simulink model "gm_uz_pmsm_model_6LUT_pd_vnl"  (R2023a)
settings: Solver=FixedStepAuto  StartTime=0.0  StopTime=0.05  RelTol=1e-3
PreLoadFcn:
  | uz_pmsm_model_init_parameter
PostLoadFcn:
  | % Import the data from Excel for a lookup table
  | FluxMapData = readtable('C:\Users\Philipp\ultrazohm\ultrazohm_sw\ip_cores\uz_pmsm_model\FluxMapData_2023-05-26_13-07-57.csv');
  | % Row indices for lookup table
  | d_current_in_d_axis = FluxMapData(8:27,1:end);
  | % Column indices for lookup table
  | q_current_in_d_axis = FluxMapData(29:48,1:end);
  | % Output values for lookup table
  | d_Flux_d_axis = FluxMapData(50:69,1:end);
undefined symbols (not defined in the file or in its folder): d_current_d_Flux, d_current_q_Flux, entkopplung_dynamic, entkopplung_linear, entkopplung_static, Flux_d, Flux_q, friction_coefficient, inertia, k_i_d, k_p_d, k_p_q, Ki_Bo_d, Ki_Bo_q, Kp_Bo_d, Kp_Bo_q, L_d, L_q, Ldd, Ldq, Lqd, Lqq, parameter_nachfuerung, polepair, praediktion_entkopplung_nonlinear, psi_pm, q_current_d_Flux, q_current_q_Flux, R_1, simulate_mechanical, simulate_nonlinear_modell, simulate_open_loop, static_friction_torque, tau_sum, ts, ts_regler
libraries: hdlmdlgenlib x5, slpidlib x4, simulink x2
(part 2 of 2)

== system gm_uz_pmsm_model_6LUT_pd_vnl/uz_pmsm_model_6LUT_vnl ==
  reset_integrators : Inport
  simulate_mechanical : Inport  Port=2
  reciprocal_J : Inport  Port=3
  mu : Inport  Port=4
  M_n0 : Inport  Port=5
  R1 : Inport  Port=6
  polepairs : Inport  Port=7
  inputs : Inport  Port=8
  Data Type Conversion{11,15..17} (4 alike) : DataTypeConversion  OutDataTypeStr=single  RndMeth=Nearest  SaturateOnIntegerOverflow=off
  Demux : Demux
  Mux : Mux
  Switch : Switch  Criteria=u2 ~= 0  SaturateOnIntegerOverflow=off  InputSameDT=off
  Switch1 : Switch  Criteria=u2 ~= 0  SaturateOnIntegerOverflow=off  InputSameDT=off
  mechanical_system : Subsystem
  pmsm : Subsystem
  torque_calculation : Subsystem
  outputs : Outport
  wires:
  Mux/1 -> outputs/1
  inputs/1 -> Demux/1
  Data Type Conversion11/1 -> Mux/1
  Data Type Conversion15/1 -> Mux/2  "i_q"
  Data Type Conversion16/1 -> Mux/3  "i_q"
  Data Type Conversion17/1 -> Mux/4  "i_q"
  pmsm/1(I_d1) -> torque_calculation/1(I_d), Data Type Conversion11/1  "i_d"
  pmsm/4(I_q1) -> Data Type Conversion15/1, torque_calculation/5(I_q)  "i_q"
  mechanical_system/1(omega_mech) -> Switch1/1, Switch/1
  Demux/2 -> pmsm/3(u_q1)  "u_q"
  M_n0/1 -> mechanical_system/4(M_n0)
  torque_calculation/1(M_Mi) -> Data Type Conversion16/1, mechanical_system/2(M_Mi)
  reciprocal_J/1 -> mechanical_system/5(reciprocal_J)
  simulate_mechanical/1 -> Switch/2, Switch1/2
  mu/1 -> mechanical_system/3(mu)
  Demux/1 -> pmsm/2(u_d1)  "u_d"
  polepairs/1 -> torque_calculation/4(polepairs), pmsm/5(polepairs1)
  pmsm/3(psi_q1) -> torque_calculation/3(psi_q)
  R1/1 -> pmsm/4(R2)
  Switch1/1 -> Data Type Conversion17/1
  Demux/4 -> mechanical_system/6(load_torque)  "load_torque"
  pmsm/2(psi_d1) -> torque_calculation/2(psi_d)
  Switch/1 -> pmsm/6(omega_mech1)
  Demux/3 -> Switch/3, Switch1/3  "omega_mech"
  reset_integrators/1 -> mechanical_system/1(reset), pmsm/1(reset1)

== system gm_uz_pmsm_model_6LUT_pd_vnl/Compare/Assert_outputs ==
  cosim : Inport
  dut : Inport  Port=2
  AssertEq : Assertion  StopWhenAssertionFail=off
  Compare To Zero : simulink/Logic and Bit Operations/Compare To Zero  relop===  OutDataTypeStr=boolean
  Constant1 : Constant  Value=0  OutDataTypeStr=Inherit: Inherit via back propagation  SampleTime=-1
  Counter : simulink/Sources/Counter Free-Running  NumBits=32  tsamp=-1
  IgnoreCycles : Constant  Value=2  OutDataTypeStr=Inherit: Inherit via back propagation  SampleTime=-1
  RelErrCheck : Subsystem
  Relational Operator : RelationalOperator  Operator=<  OutDataTypeStr=boolean  InputSameDT=off
  Switch : Switch  Criteria=u2 ~= 0  SaturateOnIntegerOverflow=off  InputSameDT=off
  Switch1 : Switch  Criteria=u2 ~= 0  SaturateOnIntegerOverflow=off  InputSameDT=off
  compare: outputs : Scope  NumInputPorts=3
  wires:
  IgnoreCycles/1 -> Relational Operator/2
  Counter/1 -> Relational Operator/1
  dut/1 -> Switch/3  "dut ref"
  cosim/1 -> Switch1/3  "cosim"
  Relational Operator/1 -> Switch1/2, Switch/2
  Constant1/1 -> Switch1/1, Switch/1
  Switch/1 -> compare: outputs/2, RelErrCheck/2(In2)
  Switch1/1 -> compare: outputs/1, RelErrCheck/1(In1)
  RelErrCheck/1(Out1) -> AssertEq/1, Compare To Zero/1  "err"
  Compare To Zero/1 -> compare: outputs/3

== system gm_uz_pmsm_model_6LUT_pd_vnl/Compare/CleanupScopes ==

== system gm_uz_pmsm_model_6LUT_pd_vnl/Compare/Enable ==

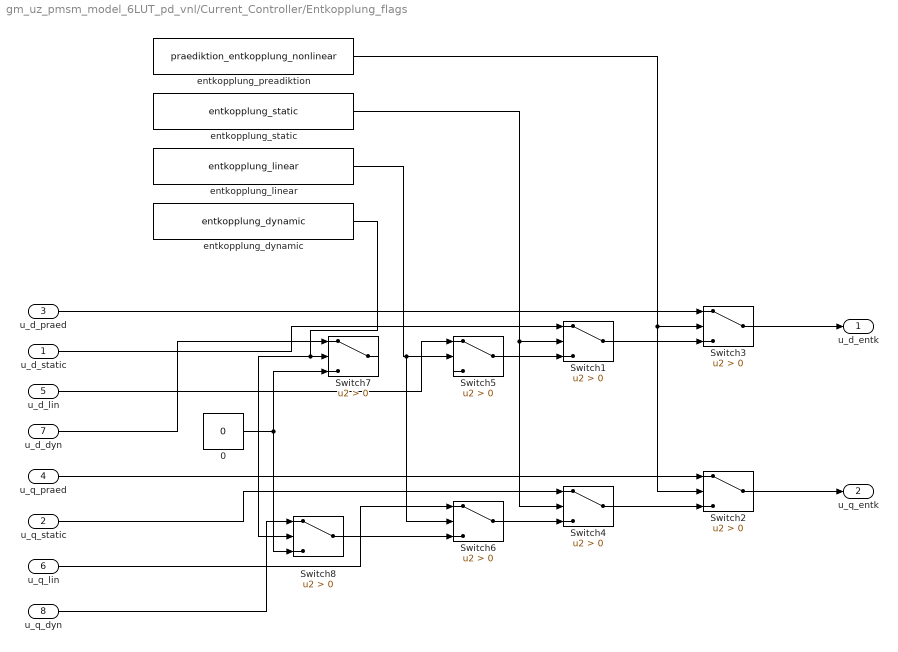
== system gm_uz_pmsm_model_6LUT_pd_vnl/Current_Controller/Entkopplung_flags ==
  u_d_static : Inport
  u_q_static : Inport  Port=2
  u_d_praed : Inport  Port=3
  u_q_praed : Inport  Port=4
  u_d_lin : Inport  Port=5
  u_q_lin : Inport  Port=6
  u_d_dyn : Inport  Port=7
  u_q_dyn : Inport  Port=8
  0 : Constant  Value=0
  Switch{1..8} (8 alike) : Switch  Criteria=u2 > Threshold  SaturateOnIntegerOverflow=off  InputSameDT=off
  entkopplung_dynamic : Constant  Value=entkopplung_dynamic
  entkopplung_linear : Constant  Value=entkopplung_linear
  entkopplung_preadiktion : Constant  Value=praediktion_entkopplung_nonlinear
  entkopplung_static : Constant  Value=entkopplung_static
  u_d_entk : Outport
  u_q_entk : Outport  Port=2
  wires:
  Switch3/1 -> u_d_entk/1
  Switch4/1 -> Switch2/3
  entkopplung_preadiktion/1 -> Switch2/2, Switch3/2
  Switch1/1 -> Switch3/3
  u_d_praed/1 -> Switch3/1
  Switch2/1 -> u_q_entk/1
  u_q_praed/1 -> Switch2/1
  entkopplung_static/1 -> Switch4/2, Switch1/2
  u_d_static/1 -> Switch1/1
  u_d_lin/1 -> Switch5/1
  Switch5/1 -> Switch1/3
  entkopplung_linear/1 -> Switch6/2, Switch5/2
  entkopplung_dynamic/1 -> Switch8/2, Switch7/2
  0/1 -> Switch8/3, Switch7/3
  Switch6/1 -> Switch4/3
  u_q_static/1 -> Switch4/1
  u_q_lin/1 -> Switch6/1
  u_d_dyn/1 -> Switch7/1
  Switch8/1 -> Switch6/3
  u_q_dyn/1 -> Switch8/1

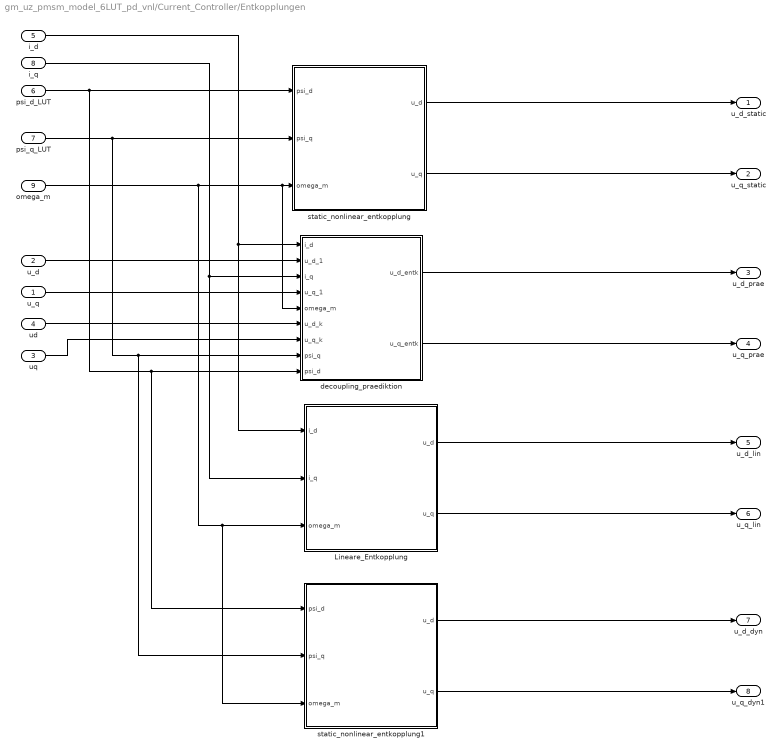
== system gm_uz_pmsm_model_6LUT_pd_vnl/Current_Controller/Entkopplungen ==
  u_q : Inport
  u_d : Inport  Port=2
  uq : Inport  Port=3
  ud : Inport  Port=4
  i_d : Inport  Port=5
  psi_d_LUT : Inport  Port=6
  psi_q_LUT : Inport  Port=7
  i_q : Inport  Port=8
  omega_m : Inport  Port=9
  Lineare_Entkopplung : Subsystem
  decoupling_praediktion : Subsystem
  static_nonlinear_entkopplung : Subsystem
  static_nonlinear_entkopplung1 : Subsystem
  u_d_static : Outport
  u_q_static : Outport  Port=2
  u_d_prae : Outport  Port=3
  u_q_prae : Outport  Port=4
  u_d_lin : Outport  Port=5
  u_q_lin : Outport  Port=6
  u_d_dyn : Outport  Port=7
  u_q_dyn1 : Outport  Port=8
  wires:
  psi_d_LUT/1 -> static_nonlinear_entkopplung/1(psi_d), static_nonlinear_entkopplung1/1(psi_d), decoupling_praediktion/9(psi_d)
  omega_m/1 -> static_nonlinear_entkopplung1/3(omega_m), Lineare_Entkopplung/3(omega_m), static_nonlinear_entkopplung/3(omega_m), decoupling_praediktion/5(omega_m)
  psi_q_LUT/1 -> static_nonlinear_entkopplung1/2(psi_q), decoupling_praediktion/8(psi_q), static_nonlinear_entkopplung/2(psi_q)
  u_q/1 -> decoupling_praediktion/4(u_q_1)
  i_d/1 -> Lineare_Entkopplung/1(i_d), decoupling_praediktion/1(i_d)
  i_q/1 -> Lineare_Entkopplung/2(i_q), decoupling_praediktion/3(i_q)
  ud/1 -> decoupling_praediktion/6(u_d_k)
  uq/1 -> decoupling_praediktion/7(u_q_k)
  u_d/1 -> decoupling_praediktion/2(u_d_1)
  static_nonlinear_entkopplung/1(u_d) -> u_d_static/1
  Lineare_Entkopplung/1(u_d) -> u_d_lin/1
  static_nonlinear_entkopplung/2(u_q) -> u_q_static/1
  decoupling_praediktion/1(u_d_entk) -> u_d_prae/1
  Lineare_Entkopplung/2(u_q) -> u_q_lin/1
  decoupling_praediktion/2(u_q_entk) -> u_q_prae/1
  static_nonlinear_entkopplung1/1(u_d) -> u_d_dyn/1
  static_nonlinear_entkopplung1/2(u_q) -> u_q_dyn1/1

== system gm_uz_pmsm_model_6LUT_pd_vnl/Current_Controller/Psi_d_q ==
  I_d_set : Inport
  I_d : Inport  Port=2
  I_q_set : Inport  Port=3
  I_q : Inport  Port=4
  Flux_d Lookup Table : Lookup_n-D  BreakpointsForDimension1=d_current_d_Flux  BreakpointsForDimension2=q_current_d_Flux  BreakpointsForDimension3=[5, 7]  Table=Flux_d  InternalRulePriority=Speed  RndMeth=Simplest
      settings: InputPortMap=u0,u1
  Flux_d Lookup Table1 : Lookup_n-D  BreakpointsForDimension1=d_current_d_Flux  BreakpointsForDimension2=q_current_d_Flux  BreakpointsForDimension3=[5, 7]  Table=Flux_d  InternalRulePriority=Speed  RndMeth=Simplest
      settings: InputPortMap=u0,u1
  Flux_q Lookup Table1 : Lookup_n-D  BreakpointsForDimension1=d_current_q_Flux  BreakpointsForDimension2=q_current_q_Flux  BreakpointsForDimension3=[5, 7]  Table=Flux_q  InternalRulePriority=Speed  RndMeth=Simplest
      settings: InputPortMap=u0,u1
  Flux_q Lookup Table2 : Lookup_n-D  BreakpointsForDimension1=d_current_q_Flux  BreakpointsForDimension2=q_current_q_Flux  BreakpointsForDimension3=[5, 7]  Table=Flux_q  InternalRulePriority=Speed  RndMeth=Simplest
      settings: InputPortMap=u0,u1
  psi_d_set : Outport
  psi_q_set : Outport  Port=2
  psi_d_LUT : Outport  Port=3
  psi_q_LUT : Outport  Port=4
  wires:
  I_d/1 -> Flux_q Lookup Table2/1, Flux_q Lookup Table1/1, Flux_d Lookup Table/1
  I_q/1 -> Flux_q Lookup Table1/2, Flux_d Lookup Table1/2, Flux_d Lookup Table/2
  I_d_set/1 -> Flux_d Lookup Table1/1
  I_q_set/1 -> Flux_q Lookup Table2/2
  Flux_d Lookup Table1/1 -> psi_d_set/1  "psi_d_set"
  Flux_q Lookup Table2/1 -> psi_q_set/1  "psi_q_set"
  Flux_d Lookup Table/1 -> psi_d_LUT/1  "psi_d_LUT"
  Flux_q Lookup Table1/1 -> psi_q_LUT/1  "psi_q_LUT"

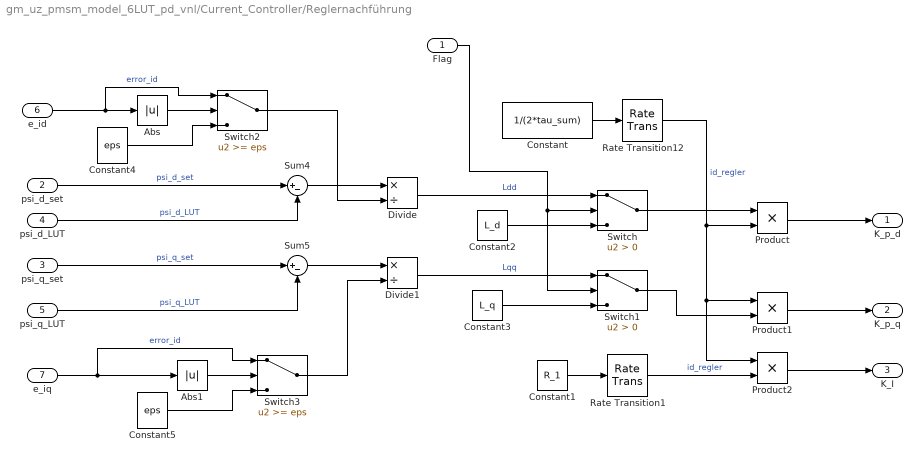
== system gm_uz_pmsm_model_6LUT_pd_vnl/Current_Controller/Reglernachführung ==
  Flag : Inport
  psi_d_set : Inport  Port=2
  psi_q_set : Inport  Port=3
  psi_d_LUT : Inport  Port=4
  psi_q_LUT : Inport  Port=5
  e_id : Inport  Port=6
  e_iq : Inport  Port=7
  Abs : Abs  SaturateOnIntegerOverflow=off
  Abs1 : Abs  SaturateOnIntegerOverflow=off
  Constant : Constant  Value=1/(2*tau_sum)
  Constant1 : Constant  Value=R_1
  Constant2 : Constant  Value=L_d
  Constant3 : Constant  Value=L_q
  Constant4 : Constant  Value=eps  SampleTime=ts_regler
  Constant5 : Constant  Value=eps  SampleTime=ts_regler
  Divide : Product  Inputs=*/
  Divide1 : Product  Inputs=*/
  Product : Product
  Product1 : Product
  Product2 : Product
  Rate Transition1 : RateTransition  OutPortSampleTime=ts_regler
  Rate Transition12 : RateTransition  OutPortSampleTime=ts_regler
  Sum4 : Sum  Inputs=|+-
  Sum5 : Sum  Inputs=|+-
  Switch : Switch  Criteria=u2 > Threshold  SaturateOnIntegerOverflow=off  InputSameDT=off
  Switch1 : Switch  Criteria=u2 > Threshold  SaturateOnIntegerOverflow=off  InputSameDT=off
  Switch2 : Switch  Threshold=eps  SaturateOnIntegerOverflow=off  InputSameDT=off
  Switch3 : Switch  Threshold=eps  SaturateOnIntegerOverflow=off  InputSameDT=off
  K_p_d : Outport
  K_p_q : Outport  Port=2
  K_I : Outport  Port=3
  wires:
  Constant/1 -> Rate Transition12/1
  Product/1 -> K_p_d/1
  Product1/1 -> K_p_q/1
  Product2/1 -> K_I/1
  Constant1/1 -> Rate Transition1/1
  Rate Transition12/1 -> Product2/1, Product1/1, Product/2  "id_regler"
  Rate Transition1/1 -> Product2/2  "id_regler"
  Flag/1 -> Switch/2, Switch1/2
  Constant2/1 -> Switch/3
  Switch/1 -> Product/1
  Constant3/1 -> Switch1/3
  Switch1/1 -> Product1/2
  Sum4/1 -> Divide/1
  psi_q_LUT/1 -> Sum5/2  "psi_q_LUT"
  Sum5/1 -> Divide1/1
  psi_d_LUT/1 -> Sum4/2  "psi_d_LUT"
  psi_d_set/1 -> Sum4/1  "psi_d_set"
  psi_q_set/1 -> Sum5/1  "psi_q_set"
  Divide/1 -> Switch/1  "Ldd"
  Divide1/1 -> Switch1/1  "Lqq"
  e_id/1 -> Switch2/1, Abs/1  "error_id"
  Constant4/1 -> Switch2/3
  Abs/1 -> Switch2/2
  Switch2/1 -> Divide/2
  e_iq/1 -> Switch3/1, Abs1/1  "error_id"
  Switch3/1 -> Divide1/2
  Abs1/1 -> Switch3/2
  Constant5/1 -> Switch3/3

== system gm_uz_pmsm_model_6LUT_pd_vnl/FOC_controller1/Psi_d_q ==
  I_d_set : Inport
  I_d : Inport  Port=2
  I_q_set : Inport  Port=3
  I_q : Inport  Port=4
  Flux_d Lookup Table : Lookup_n-D  BreakpointsForDimension1=d_current_d_Flux  BreakpointsForDimension2=q_current_d_Flux  BreakpointsForDimension3=[5, 7]  Table=Flux_d  InternalRulePriority=Speed  RndMeth=Simplest
      settings: InputPortMap=u0,u1
  Flux_d Lookup Table1 : Lookup_n-D  BreakpointsForDimension1=d_current_d_Flux  BreakpointsForDimension2=q_current_d_Flux  BreakpointsForDimension3=[5, 7]  Table=Flux_d  InternalRulePriority=Speed  RndMeth=Simplest
      settings: InputPortMap=u0,u1
  Flux_q Lookup Table1 : Lookup_n-D  BreakpointsForDimension1=d_current_q_Flux  BreakpointsForDimension2=q_current_q_Flux  BreakpointsForDimension3=[5, 7]  Table=Flux_q  InternalRulePriority=Speed  RndMeth=Simplest
      settings: InputPortMap=u0,u1
  Flux_q Lookup Table2 : Lookup_n-D  BreakpointsForDimension1=d_current_q_Flux  BreakpointsForDimension2=q_current_q_Flux  BreakpointsForDimension3=[5, 7]  Table=Flux_q  InternalRulePriority=Speed  RndMeth=Simplest
      settings: InputPortMap=u0,u1
  psi_d_set : Outport
  psi_q_set : Outport  Port=2
  psi_d_LUT : Outport  Port=3
  psi_q_LUT : Outport  Port=4
  wires:
  I_d/1 -> Flux_q Lookup Table2/1, Flux_q Lookup Table1/1, Flux_d Lookup Table/1
  I_q/1 -> Flux_q Lookup Table1/2, Flux_d Lookup Table1/2, Flux_d Lookup Table/2
  I_d_set/1 -> Flux_d Lookup Table1/1
  I_q_set/1 -> Flux_q Lookup Table2/2
  Flux_d Lookup Table1/1 -> psi_d_set/1  "psi_d_set"
  Flux_q Lookup Table2/1 -> psi_q_set/1  "psi_q_set"
  Flux_d Lookup Table/1 -> psi_d_LUT/1  "psi_d_LUT"
  Flux_q Lookup Table1/1 -> psi_q_LUT/1  "psi_q_LUT"

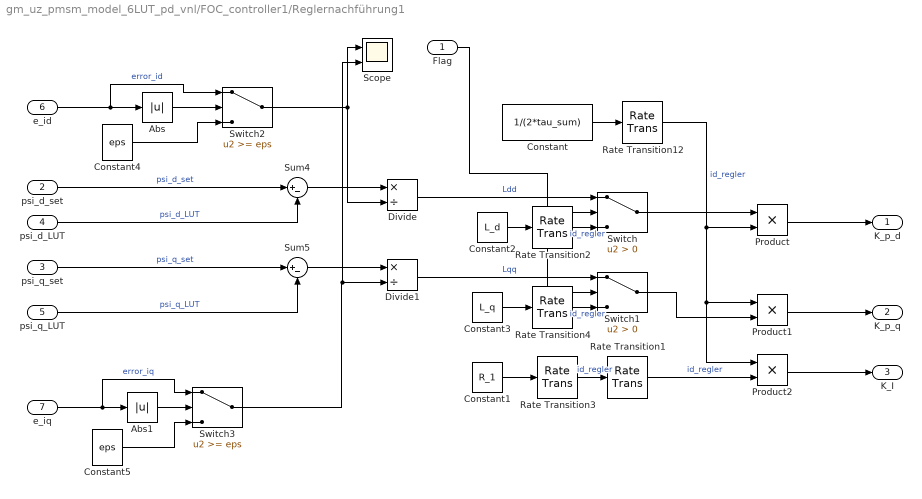
== system gm_uz_pmsm_model_6LUT_pd_vnl/FOC_controller1/Reglernachführung1 ==
  Flag : Inport
  psi_d_set : Inport  Port=2
  psi_q_set : Inport  Port=3
  psi_d_LUT : Inport  Port=4
  psi_q_LUT : Inport  Port=5
  e_id : Inport  Port=6
  e_iq : Inport  Port=7
  Abs : Abs  SaturateOnIntegerOverflow=off
  Abs1 : Abs  SaturateOnIntegerOverflow=off
  Constant : Constant  Value=1/(2*tau_sum)
  Constant1 : Constant  Value=R_1
  Constant2 : Constant  Value=L_d
  Constant3 : Constant  Value=L_q
  Constant4 : Constant  Value=eps  SampleTime=ts_regler
  Constant5 : Constant  Value=eps  SampleTime=ts_regler
  Divide : Product  Inputs=*/
  Divide1 : Product  Inputs=*/
  Product : Product
  Product1 : Product
  Product2 : Product
  Rate Transition{1..4,12} (5 alike) : RateTransition  OutPortSampleTime=ts_regler
  Scope : Scope  NumInputPorts=2
  Sum4 : Sum  Inputs=|+-
  Sum5 : Sum  Inputs=|+-
  Switch : Switch  Criteria=u2 > Threshold  SaturateOnIntegerOverflow=off  InputSameDT=off
  Switch1 : Switch  Criteria=u2 > Threshold  SaturateOnIntegerOverflow=off  InputSameDT=off
  Switch2 : Switch  Threshold=eps  SaturateOnIntegerOverflow=off  InputSameDT=off
  Switch3 : Switch  Threshold=eps  SaturateOnIntegerOverflow=off  InputSameDT=off
  K_p_d : Outport
  K_p_q : Outport  Port=2
  K_I : Outport  Port=3
  wires:
  Constant/1 -> Rate Transition12/1
  Product/1 -> K_p_d/1
  Product1/1 -> K_p_q/1
  Product2/1 -> K_I/1
  Constant1/1 -> Rate Transition3/1
  Rate Transition12/1 -> Product2/1, Product1/1, Product/2  "id_regler"
  Rate Transition1/1 -> Product2/2  "id_regler"
  Flag/1 -> Switch/2, Switch1/2
  Constant2/1 -> Rate Transition2/1
  Switch/1 -> Product/1
  Constant3/1 -> Rate Transition4/1
  Switch1/1 -> Product1/2
  e_id/1 -> Switch2/1, Abs/1  "error_id"
  e_iq/1 -> Switch3/1, Abs1/1  "error_iq"
  Sum4/1 -> Divide/1
  Abs1/1 -> Switch3/2
  psi_q_LUT/1 -> Sum5/2  "psi_q_LUT"
  Sum5/1 -> Divide1/1
  psi_d_LUT/1 -> Sum4/2  "psi_d_LUT"
  psi_d_set/1 -> Sum4/1  "psi_d_set"
  psi_q_set/1 -> Sum5/1  "psi_q_set"
  Divide/1 -> Switch/1  "Ldd"
  Divide1/1 -> Switch1/1  "Lqq"
  Abs/1 -> Switch2/2
  Constant4/1 -> Switch2/3
  Switch2/1 -> Scope/1, Divide/2
  Constant5/1 -> Switch3/3
  Switch3/1 -> Scope/2, Divide1/2
  Rate Transition2/1 -> Switch/3  "id_regler"
  Rate Transition3/1 -> Rate Transition1/1  "id_regler"
  Rate Transition4/1 -> Switch1/3  "id_regler"

== system gm_uz_pmsm_model_6LUT_pd_vnl/FOC_controller1/decoupling2 ==
  i_d : Inport
  i_q : Inport  Port=2
  omega_m : Inport  Port=3
  Flux_d Lookup Table : Lookup_n-D  BreakpointsForDimension1=d_current_d_Flux  BreakpointsForDimension2=q_current_d_Flux  BreakpointsForDimension3=[5, 7]  Table=Flux_d  InternalRulePriority=Speed  RndMeth=Simplest
      settings: InputPortMap=u0,u1
  Flux_q Lookup Table1 : Lookup_n-D  BreakpointsForDimension1=d_current_q_Flux  BreakpointsForDimension2=q_current_q_Flux  BreakpointsForDimension3=[5, 7]  Table=Flux_q  InternalRulePriority=Speed  RndMeth=Simplest
      settings: InputPortMap=u0,u1
  Gain2 : Gain  Gain=polepair
  Product : Product
  Product1 : Product
  Scope : Scope  NumInputPorts=2
  u_d : Outport
  u_q : Outport  Port=2
  wires:
  Flux_d Lookup Table/1 -> Product/1
  Gain2/1 -> Product1/2, Product/2
  Product1/1 -> Scope/1, u_q/1
  i_d/1 -> Flux_q Lookup Table1/1, Flux_d Lookup Table/1
  Product/1 -> Scope/2, u_d/1
  i_q/1 -> Flux_q Lookup Table1/2, Flux_d Lookup Table/2
  Flux_q Lookup Table1/1 -> Product1/1
  omega_m/1 -> Gain2/1

== system gm_uz_pmsm_model_6LUT_pd_vnl/pmsm/Subsystem ==
  in : Inport
  reset : Inport  Port=2
  Delay1 : Delay  DelayLength=1  ExternalReset=Level
      settings: InputPortMap=u0,r5
  Gain7 : Gain  Gain=ts  OutDataTypeStr=double
  Sum5 : Sum  Inputs=|++  OutDataTypeStr=double
  outt : Outport
  wires:
  in/1 -> Gain7/1
  reset/1 -> Delay1/2
  Delay1/1 -> outt/1, Sum5/2
  Gain7/1 -> Sum5/1
  Sum5/1 -> Delay1/1

== system gm_uz_pmsm_model_6LUT_pd_vnl/pmsm/Subsystem1 ==
  in : Inport
  reset : Inport  Port=2
  Delay1 : Delay  DelayLength=1  ExternalReset=Level
      settings: InputPortMap=u0,r5
  Gain7 : Gain  Gain=ts  OutDataTypeStr=double
  Sum5 : Sum  Inputs=|++  OutDataTypeStr=double
  outt : Outport
  wires:
  in/1 -> Gain7/1
  reset/1 -> Delay1/2
  Delay1/1 -> outt/1, Sum5/2
  Gain7/1 -> Sum5/1
  Sum5/1 -> Delay1/1

== system gm_uz_pmsm_model_6LUT_pd_vnl/uz_pmsm_model_6LUT/Abs ==
  In1 : Inport
  Abs : Abs  SampleTime=1e-08  OutDataTypeStr=single  SaturateOnIntegerOverflow=off
  Out1 : Outport
  wires:
  Abs/1 -> Out1/1
  In1/1 -> Abs/1

== system gm_uz_pmsm_model_6LUT_pd_vnl/uz_pmsm_model_6LUT/Divide ==
  In1 : Inport
  In2 : Inport  Port=2
  Divide : Product  Inputs=**  OutDataTypeStr=single  SampleTime=1e-08
  Divide_pd1 : Delay  DelayLength=6
  Out1 : Outport
  wires:
  Divide_pd1/1 -> Out1/1
  Divide/1 -> Divide_pd1/1
  In2/1 -> Divide/2
  In1/1 -> Divide/1

== system gm_uz_pmsm_model_6LUT_pd_vnl/uz_pmsm_model_6LUT/Divide1 ==
  In1 : Inport
  In2 : Inport  Port=2
  Divide1 : Product  Inputs=*/  OutDataTypeStr=single  SampleTime=1e-08
  Divide1_pd1 : Delay  DelayLength=17
  Out1 : Outport
  wires:
  Divide1_pd1/1 -> Out1/1
  Divide1/1 -> Divide1_pd1/1
  In2/1 -> Divide1/2
  In1/1 -> Divide1/1

== system gm_uz_pmsm_model_6LUT_pd_vnl/uz_pmsm_model_6LUT/Divide_recip ==
  In1 : Inport
  Divide_recip : Math  Operator=reciprocal  SampleTime=1e-08
  Divide_recip_pd1 : Delay  DelayLength=16
  Out1 : Outport
  wires:
  Divide_recip_pd1/1 -> Out1/1
  Divide_recip/1 -> Divide_recip_pd1/1
  In1/1 -> Divide_recip/1

== system gm_uz_pmsm_model_6LUT_pd_vnl/uz_pmsm_model_6LUT/Factor ==
  In1 : Inport
  In2 : Inport  Port=2
  Factor : Product  Inputs=**  OutDataTypeStr=single  SampleTime=1e-08
  Factor_pd1 : Delay  DelayLength=6
  Out1 : Outport
  wires:
  Factor_pd1/1 -> Out1/1
  Factor/1 -> Factor_pd1/1
  In2/1 -> Factor/2
  In1/1 -> Factor/1

== system gm_uz_pmsm_model_6LUT_pd_vnl/uz_pmsm_model_6LUT/Flux_d Lookup Table ==
  In1 : Inport
  In2 : Inport  Port=2
  Flux_d Lookup Table : Lookup_n-D  BreakpointsForDimension1=d_current_q_Flux  BreakpointsForDimension2=q_current_q_Flux  BreakpointsForDimension3=[5, 7]  Table=Flux_d  ExtrapMethod=Clip  UseLastTableValue=on  InternalRulePriority=Speed  OutDataTypeStr=Inherit: Inherit from 'Table data'  RndMeth=Simplest
      settings: InputPortMap=u0,u1
  Flux_d Lookup Table_pd1 : Delay  DelayLength=53
  Out1 : Outport
  wires:
  In2/1 -> Flux_d Lookup Table/2
  In1/1 -> Flux_d Lookup Table/1
  Flux_d Lookup Table/1 -> Flux_d Lookup Table_pd1/1
  Flux_d Lookup Table_pd1/1 -> Out1/1

== system gm_uz_pmsm_model_6LUT_pd_vnl/uz_pmsm_model_6LUT/Flux_q Lookup Table ==
  In1 : Inport
  In2 : Inport  Port=2
  Flux_q Lookup Table : Lookup_n-D  BreakpointsForDimension1=d_current_q_Flux  BreakpointsForDimension2=q_current_q_Flux  BreakpointsForDimension3=[5, 7]  Table=Flux_q  ExtrapMethod=Clip  UseLastTableValue=on  InternalRulePriority=Speed  OutDataTypeStr=Inherit: Inherit from 'Table data'  RndMeth=Simplest
      settings: InputPortMap=u0,u1
  Flux_q Lookup Table_pd1 : Delay  DelayLength=53
  Out1 : Outport
  wires:
  In2/1 -> Flux_q Lookup Table/2
  In1/1 -> Flux_q Lookup Table/1
  Flux_q Lookup Table/1 -> Flux_q Lookup Table_pd1/1
  Flux_q Lookup Table_pd1/1 -> Out1/1

== system gm_uz_pmsm_model_6LUT_pd_vnl/uz_pmsm_model_6LUT/Gain ==
  In1 : Inport
  In2 : Inport  Port=2
  Gain : Product  Inputs=**  OutDataTypeStr=single  SampleTime=1e-08
  Gain_pd1 : Delay  DelayLength=6
  Out1 : Outport
  wires:
  Gain_pd1/1 -> Out1/1
  Gain/1 -> Gain_pd1/1
  In2/1 -> Gain/2
  In1/1 -> Gain/1

== system gm_uz_pmsm_model_6LUT_pd_vnl/uz_pmsm_model_6LUT/Gain7 ==
  In1 : Inport
  In2 : Inport  Port=2
  Gain7 : Product  Inputs=**  OutDataTypeStr=single  SampleTime=1e-08
  Gain7_pd1 : Delay  DelayLength=6
  Out1 : Outport
  wires:
  Gain7_pd1/1 -> Out1/1
  Gain7/1 -> Gain7_pd1/1
  In2/1 -> Gain7/2
  In1/1 -> Gain7/1

== system gm_uz_pmsm_model_6LUT_pd_vnl/uz_pmsm_model_6LUT/Gain71 ==
  In1 : Inport
  In2 : Inport  Port=2
  Gain71 : Product  Inputs=**  OutDataTypeStr=single  SampleTime=1e-08
  Gain71_pd1 : Delay  DelayLength=6
  Out1 : Outport
  wires:
  Gain71_pd1/1 -> Out1/1
  Gain71/1 -> Gain71_pd1/1
  In2/1 -> Gain71/2
  In1/1 -> Gain71/1

== system gm_uz_pmsm_model_6LUT_pd_vnl/uz_pmsm_model_6LUT/Ldd Lookup Table ==
  In1 : Inport
  In2 : Inport  Port=2
  Ldd Lookup Table : Lookup_n-D  BreakpointsForDimension1=d_current_q_Flux  BreakpointsForDimension2=q_current_q_Flux  BreakpointsForDimension3=[5, 7]  Table=Ldd  ExtrapMethod=Clip  UseLastTableValue=on  InternalRulePriority=Speed  OutDataTypeStr=Inherit: Inherit from 'Table data'  RndMeth=Simplest
      settings: InputPortMap=u0,u1
  Ldd Lookup Table_pd1 : Delay  DelayLength=53
  Out1 : Outport
  wires:
  Ldd Lookup Table_pd1/1 -> Out1/1
  Ldd Lookup Table/1 -> Ldd Lookup Table_pd1/1
  In1/1 -> Ldd Lookup Table/1
  In2/1 -> Ldd Lookup Table/2

== system gm_uz_pmsm_model_6LUT_pd_vnl/uz_pmsm_model_6LUT/Ldq Lookup Table2 ==
  In1 : Inport
  In2 : Inport  Port=2
  Ldq Lookup Table2 : Lookup_n-D  BreakpointsForDimension1=d_current_q_Flux  BreakpointsForDimension2=q_current_q_Flux  BreakpointsForDimension3=[5, 7]  Table=Ldq  ExtrapMethod=Clip  UseLastTableValue=on  InternalRulePriority=Speed  OutDataTypeStr=Inherit: Inherit from 'Table data'  RndMeth=Simplest
      settings: InputPortMap=u0,u1
  Ldq Lookup Table2_pd1 : Delay  DelayLength=53
  Out1 : Outport
  wires:
  In1/1 -> Ldq Lookup Table2/1
  In2/1 -> Ldq Lookup Table2/2
  Ldq Lookup Table2/1 -> Ldq Lookup Table2_pd1/1
  Ldq Lookup Table2_pd1/1 -> Out1/1

== system gm_uz_pmsm_model_6LUT_pd_vnl/uz_pmsm_model_6LUT/Lqd Lookup Table1 ==
  In1 : Inport
  In2 : Inport  Port=2
  Lqd Lookup Table1 : Lookup_n-D  BreakpointsForDimension1=d_current_q_Flux  BreakpointsForDimension2=q_current_q_Flux  BreakpointsForDimension3=[5, 7]  Table=Lqd  ExtrapMethod=Clip  UseLastTableValue=on  InternalRulePriority=Speed  OutDataTypeStr=Inherit: Inherit from 'Table data'  RndMeth=Simplest
      settings: InputPortMap=u0,u1
  Lqd Lookup Table1_pd1 : Delay  DelayLength=53
  Out1 : Outport
  wires:
  In1/1 -> Lqd Lookup Table1/1
  In2/1 -> Lqd Lookup Table1/2
  Lqd Lookup Table1/1 -> Lqd Lookup Table1_pd1/1
  Lqd Lookup Table1_pd1/1 -> Out1/1

== system gm_uz_pmsm_model_6LUT_pd_vnl/uz_pmsm_model_6LUT/Lqq Lookup Table ==
  In1 : Inport
  In2 : Inport  Port=2
  Lqq Lookup Table : Lookup_n-D  BreakpointsForDimension1=d_current_q_Flux  BreakpointsForDimension2=q_current_q_Flux  BreakpointsForDimension3=[5, 7]  Table=Lqq  ExtrapMethod=Clip  UseLastTableValue=on  InternalRulePriority=Speed  OutDataTypeStr=Inherit: Inherit from 'Table data'  RndMeth=Simplest
      settings: InputPortMap=u0,u1
  Lqq Lookup Table_pd1 : Delay  DelayLength=53
  Out1 : Outport
  wires:
  Lqq Lookup Table/1 -> Lqq Lookup Table_pd1/1
  In2/1 -> Lqq Lookup Table/2
  Lqq Lookup Table_pd1/1 -> Out1/1
  In1/1 -> Lqq Lookup Table/1

== system gm_uz_pmsm_model_6LUT_pd_vnl/uz_pmsm_model_6LUT/Product11 ==
  In1 : Inport
  In2 : Inport  Port=2
  Product11 : Product  Inputs=**  OutDataTypeStr=single  SampleTime=1e-08
  Product11_pd1 : Delay  DelayLength=6
  Out1 : Outport
  wires:
  Product11_pd1/1 -> Out1/1
  Product11/1 -> Product11_pd1/1
  In2/1 -> Product11/2
  In1/1 -> Product11/1

== system gm_uz_pmsm_model_6LUT_pd_vnl/uz_pmsm_model_6LUT/Product111 ==
  In1 : Inport
  In2 : Inport  Port=2
  Product111 : Product  Inputs=**  OutDataTypeStr=single  SampleTime=1e-08
  Product111_pd1 : Delay  DelayLength=6
  Out1 : Outport
  wires:
  Product111_pd1/1 -> Out1/1
  Product111/1 -> Product111_pd1/1
  In2/1 -> Product111/2
  In1/1 -> Product111/1

== system gm_uz_pmsm_model_6LUT_pd_vnl/uz_pmsm_model_6LUT/Product12 ==
  In1 : Inport
  In2 : Inport  Port=2
  Product12 : Product  Inputs=**  OutDataTypeStr=single  SampleTime=1e-08
  Product12_pd1 : Delay  DelayLength=6
  Out1 : Outport
  wires:
  Product12_pd1/1 -> Out1/1
  Product12/1 -> Product12_pd1/1
  In2/1 -> Product12/2
  In1/1 -> Product12/1

== system gm_uz_pmsm_model_6LUT_pd_vnl/uz_pmsm_model_6LUT/Product121 ==
  In1 : Inport
  In2 : Inport  Port=2
  Product121 : Product  Inputs=**  OutDataTypeStr=single  SampleTime=1e-08
  Product121_pd1 : Delay  DelayLength=6
  Out1 : Outport
  wires:
  Product121_pd1/1 -> Out1/1
  Product121/1 -> Product121_pd1/1
  In2/1 -> Product121/2
  In1/1 -> Product121/1

== system gm_uz_pmsm_model_6LUT_pd_vnl/uz_pmsm_model_6LUT/Product13 ==
  In1 : Inport
  In2 : Inport  Port=2
  Product13 : Product  Inputs=**  OutDataTypeStr=single  SampleTime=1e-08
  Product13_pd1 : Delay  DelayLength=6
  Out1 : Outport
  wires:
  Product13_pd1/1 -> Out1/1
  Product13/1 -> Product13_pd1/1
  In2/1 -> Product13/2
  In1/1 -> Product13/1

== system gm_uz_pmsm_model_6LUT_pd_vnl/uz_pmsm_model_6LUT/Product2 ==
  In1 : Inport
  In2 : Inport  Port=2
  Product2 : Product  Inputs=**  OutDataTypeStr=single  SampleTime=1e-08
  Product2_pd1 : Delay  DelayLength=6
  Out1 : Outport
  wires:
  Product2_pd1/1 -> Out1/1
  Product2/1 -> Product2_pd1/1
  In2/1 -> Product2/2
  In1/1 -> Product2/1

== system gm_uz_pmsm_model_6LUT_pd_vnl/uz_pmsm_model_6LUT/Product21 ==
  In1 : Inport
  In2 : Inport  Port=2
  Product21 : Product  Inputs=**  OutDataTypeStr=single  SampleTime=1e-08
  Product21_pd1 : Delay  DelayLength=6
  Out1 : Outport
  wires:
  Product21_pd1/1 -> Out1/1
  Product21/1 -> Product21_pd1/1
  In2/1 -> Product21/2
  In1/1 -> Product21/1

== system gm_uz_pmsm_model_6LUT_pd_vnl/uz_pmsm_model_6LUT/Product3 ==
  In1 : Inport
  In2 : Inport  Port=2
  Product3 : Product  Inputs=**  OutDataTypeStr=single  SampleTime=1e-08
  Product3_pd1 : Delay  DelayLength=6
  Out1 : Outport
  wires:
  Product3_pd1/1 -> Out1/1
  Product3/1 -> Product3_pd1/1
  In2/1 -> Product3/2
  In1/1 -> Product3/1

== system gm_uz_pmsm_model_6LUT_pd_vnl/uz_pmsm_model_6LUT/Product31 ==
  In1 : Inport
  In2 : Inport  Port=2
  Product31 : Product  Inputs=**  OutDataTypeStr=single  SampleTime=1e-08
  Product31_pd1 : Delay  DelayLength=6
  Out1 : Outport
  wires:
  Product31_pd1/1 -> Out1/1
  Product31/1 -> Product31_pd1/1
  In2/1 -> Product31/2
  In1/1 -> Product31/1

== system gm_uz_pmsm_model_6LUT_pd_vnl/uz_pmsm_model_6LUT/Product4 ==
  In1 : Inport
  In2 : Inport  Port=2
  Product4 : Product  Inputs=**  OutDataTypeStr=single  SampleTime=1e-08
  Product4_pd1 : Delay  DelayLength=6
  Out1 : Outport
  wires:
  Product4_pd1/1 -> Out1/1
  Product4/1 -> Product4_pd1/1
  In2/1 -> Product4/2
  In1/1 -> Product4/1

== system gm_uz_pmsm_model_6LUT_pd_vnl/uz_pmsm_model_6LUT/Product41 ==
  In1 : Inport
  In2 : Inport  Port=2
  Product41 : Product  Inputs=**  OutDataTypeStr=single  SampleTime=1e-08
  Product41_pd1 : Delay  DelayLength=6
  Out1 : Outport
  wires:
  Product41_pd1/1 -> Out1/1
  Product41/1 -> Product41_pd1/1
  In2/1 -> Product41/2
  In1/1 -> Product41/1

== system gm_uz_pmsm_model_6LUT_pd_vnl/uz_pmsm_model_6LUT/Product9 ==
  In1 : Inport
  In2 : Inport  Port=2
  Product9 : Product  Inputs=**  OutDataTypeStr=single  SampleTime=1e-08
  Product9_pd1 : Delay  DelayLength=6
  Out1 : Outport
  wires:
  Product9_pd1/1 -> Out1/1
  Product9/1 -> Product9_pd1/1
  In2/1 -> Product9/2
  In1/1 -> Product9/1

== system gm_uz_pmsm_model_6LUT_pd_vnl/uz_pmsm_model_6LUT/Product91 ==
  In1 : Inport
  In2 : Inport  Port=2
  Product91 : Product  Inputs=**  OutDataTypeStr=single  SampleTime=1e-08
  Product91_pd1 : Delay  DelayLength=6
  Out1 : Outport
  wires:
  Product91_pd1/1 -> Out1/1
  Product91/1 -> Product91_pd1/1
  In2/1 -> Product91/2
  In1/1 -> Product91/1

== system gm_uz_pmsm_model_6LUT_pd_vnl/uz_pmsm_model_6LUT/Sign1 ==
  In1 : Inport
  Sign1 : Signum  SampleTime=1e-08
  Out1 : Outport
  wires:
  Sign1/1 -> Out1/1
  In1/1 -> Sign1/1

== system gm_uz_pmsm_model_6LUT_pd_vnl/uz_pmsm_model_6LUT/Sum ==
  In1 : Inport
  In2 : Inport  Port=2
  Sum : Sum  Inputs=+-  OutDataTypeStr=single  SampleTime=1e-08
  Sum_pd1 : Delay  DelayLength=6
  Out1 : Outport
  wires:
  Sum_pd1/1 -> Out1/1
  Sum/1 -> Sum_pd1/1
  In2/1 -> Sum/2
  In1/1 -> Sum/1

== system gm_uz_pmsm_model_6LUT_pd_vnl/uz_pmsm_model_6LUT/Sum1 ==
  In1 : Inport
  In2 : Inport  Port=2
  Sum1 : Sum  Inputs=+-  OutDataTypeStr=single  SampleTime=1e-08
  Sum1_pd1 : Delay  DelayLength=6
  Out1 : Outport
  wires:
  Sum1_pd1/1 -> Out1/1
  Sum1/1 -> Sum1_pd1/1
  In2/1 -> Sum1/2
  In1/1 -> Sum1/1

== system gm_uz_pmsm_model_6LUT_pd_vnl/uz_pmsm_model_6LUT/Sum3 ==
  In1 : Inport
  In2 : Inport  Port=2
  Sum3 : Sum  OutDataTypeStr=single  SampleTime=1e-08
  Sum3_pd1 : Delay  DelayLength=6
  Out1 : Outport
  wires:
  Sum3_pd1/1 -> Out1/1
  Sum3/1 -> Sum3_pd1/1
  In2/1 -> Sum3/2
  In1/1 -> Sum3/1

== system gm_uz_pmsm_model_6LUT_pd_vnl/uz_pmsm_model_6LUT/Sum31 ==
  In1 : Inport
  In2 : Inport  Port=2
  Sum31 : Sum  Inputs=+-  OutDataTypeStr=single  SampleTime=1e-08
  Sum31_pd1 : Delay  DelayLength=6
  Out1 : Outport
  wires:
  Sum31_pd1/1 -> Out1/1
  Sum31/1 -> Sum31_pd1/1
  In2/1 -> Sum31/2
  In1/1 -> Sum31/1

== system gm_uz_pmsm_model_6LUT_pd_vnl/uz_pmsm_model_6LUT/Sum3_stage2 ==
  In1 : Inport
  In2 : Inport  Port=2
  Sum3_stage2 : Sum  Inputs=+-  OutDataTypeStr=single  SampleTime=1e-08
  Sum3_stage2_pd1 : Delay  DelayLength=6
  Out1 : Outport
  wires:
  Sum3_stage2_pd1/1 -> Out1/1
  Sum3_stage2/1 -> Sum3_stage2_pd1/1
  In2/1 -> Sum3_stage2/2
  In1/1 -> Sum3_stage2/1

== system gm_uz_pmsm_model_6LUT_pd_vnl/uz_pmsm_model_6LUT/Sum3_stage3 ==
  In1 : Inport
  In2 : Inport  Port=2
  Sum3_stage3 : Sum  Inputs=+-  OutDataTypeStr=single  SampleTime=1e-08
  Sum3_stage3_pd1 : Delay  DelayLength=6
  Out1 : Outport
  wires:
  Sum3_stage3_pd1/1 -> Out1/1
  Sum3_stage3/1 -> Sum3_stage3_pd1/1
  In2/1 -> Sum3_stage3/2
  In1/1 -> Sum3_stage3/1

== system gm_uz_pmsm_model_6LUT_pd_vnl/uz_pmsm_model_6LUT/Sum3_stage4 ==
  In1 : Inport
  In2 : Inport  Port=2
  Sum3_stage4 : Sum  OutDataTypeStr=single  SampleTime=1e-08
  Sum3_stage4_pd1 : Delay  DelayLength=6
  Out1 : Outport
  wires:
  Sum3_stage4_pd1/1 -> Out1/1
  Sum3_stage4/1 -> Sum3_stage4_pd1/1
  In2/1 -> Sum3_stage4/2
  In1/1 -> Sum3_stage4/1

== system gm_uz_pmsm_model_6LUT_pd_vnl/uz_pmsm_model_6LUT/Sum4_stage2 ==
  In1 : Inport
  In2 : Inport  Port=2
  Sum4_stage2 : Sum  Inputs=+-  OutDataTypeStr=single  SampleTime=1e-08
  Sum4_stage2_pd1 : Delay  DelayLength=6
  Out1 : Outport
  wires:
  Sum4_stage2_pd1/1 -> Out1/1
  Sum4_stage2/1 -> Sum4_stage2_pd1/1
  In2/1 -> Sum4_stage2/2
  In1/1 -> Sum4_stage2/1

== system gm_uz_pmsm_model_6LUT_pd_vnl/uz_pmsm_model_6LUT/Sum4_stage3 ==
  In1 : Inport
  In2 : Inport  Port=2
  Sum4_stage3 : Sum  Inputs=+-  OutDataTypeStr=single  SampleTime=1e-08
  Sum4_stage3_pd1 : Delay  DelayLength=6
  Out1 : Outport
  wires:
  Sum4_stage3_pd1/1 -> Out1/1
  Sum4_stage3/1 -> Sum4_stage3_pd1/1
  In2/1 -> Sum4_stage3/2
  In1/1 -> Sum4_stage3/1

== system gm_uz_pmsm_model_6LUT_pd_vnl/uz_pmsm_model_6LUT/Sum4_stage4 ==
  In1 : Inport
  In2 : Inport  Port=2
  Sum4_stage4 : Sum  Inputs=+-  OutDataTypeStr=single  SampleTime=1e-08
  Sum4_stage4_pd1 : Delay  DelayLength=6
  Out1 : Outport
  wires:
  Sum4_stage4_pd1/1 -> Out1/1
  Sum4_stage4/1 -> Sum4_stage4_pd1/1
  In2/1 -> Sum4_stage4/2
  In1/1 -> Sum4_stage4/1

== system gm_uz_pmsm_model_6LUT_pd_vnl/uz_pmsm_model_6LUT/Sum5 ==
  In1 : Inport
  In2 : Inport  Port=2
  Sum5 : Sum  OutDataTypeStr=single  SampleTime=1e-08
  Sum5_pd1 : Delay  DelayLength=6
  Out1 : Outport
  wires:
  Sum5_pd1/1 -> Out1/1
  Sum5/1 -> Sum5_pd1/1
  In2/1 -> Sum5/2
  In1/1 -> Sum5/1

== system gm_uz_pmsm_model_6LUT_pd_vnl/uz_pmsm_model_6LUT/Sum51 ==
  In1 : Inport
  In2 : Inport  Port=2
  Sum51 : Sum  OutDataTypeStr=single  SampleTime=1e-08
  Sum51_pd1 : Delay  DelayLength=6
  Out1 : Outport
  wires:
  Sum51_pd1/1 -> Out1/1
  Sum51/1 -> Sum51_pd1/1
  In2/1 -> Sum51/2
  In1/1 -> Sum51/1

== system gm_uz_pmsm_model_6LUT_pd_vnl/uz_pmsm_model_6LUT/Sum52 ==
  In1 : Inport
  In2 : Inport  Port=2
  Sum52 : Sum  OutDataTypeStr=single  SampleTime=1e-08
  Sum52_pd1 : Delay  DelayLength=6
  Out1 : Outport
  wires:
  Sum52_pd1/1 -> Out1/1
  Sum52/1 -> Sum52_pd1/1
  In2/1 -> Sum52/2
  In1/1 -> Sum52/1

== system gm_uz_pmsm_model_6LUT_pd_vnl/uz_pmsm_model_6LUT_vnl/mechanical_system ==
  note: This delay breaks the algebraic loop between mechanical and electrical system.
      | Introduces a delay of 500ns.
  reset : Inport
  M_Mi : Inport  Port=2
  mu : Inport  Port=3
  M_n0 : Inport  Port=4
  reciprocal_J : Inport  Port=5
  load_torque : Inport  Port=6
  Abs : Abs  SaturateOnIntegerOverflow=off
  Delay : Delay  DelayLength=1
  Product11 : Product
  Product12 : Product
  Product4 : Product
  Sign1 : Signum
  Sum : Sum  Inputs=|+-  OutDataTypeStr=single
  Sum1 : Sum  Inputs=|+-
  Sum5 : Sum  Inputs=|++
  integrator1 : Subsystem
  omega_mech : Outport
  wires:
  Delay/1 -> Sum1/1
  Product4/1 -> Sum/2
  Sum/1 -> Delay/1
  load_torque/1 -> Sum1/2
  Sum1/1 -> Product11/2
  M_Mi/1 -> Sum/1
  reciprocal_J/1 -> Product11/1
  M_n0/1 -> Sum5/2
  mu/1 -> Product12/1
  Product12/1 -> Sum5/1
  reset/1 -> integrator1/1(reset)
  Abs/1 -> Product12/2
  integrator1/1(outt) -> omega_mech/1, Abs/1, Sign1/1
  Sign1/1 -> Product4/2
  Sum5/1 -> Product4/1
  Product11/1 -> integrator1/2(in)

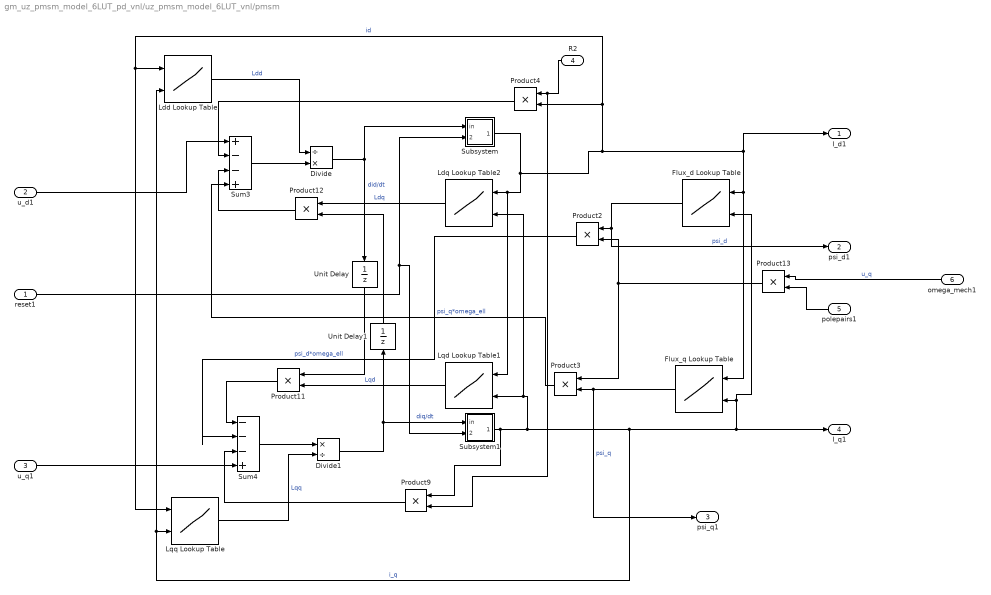
== system gm_uz_pmsm_model_6LUT_pd_vnl/uz_pmsm_model_6LUT_vnl/pmsm ==
  reset1 : Inport
  u_d1 : Inport  Port=2
  u_q1 : Inport  Port=3
  R2 : Inport  Port=4
  polepairs1 : Inport  Port=5
  omega_mech1 : Inport  Port=6
  Divide : Product  Inputs=/*  OutDataTypeStr=single
  Divide1 : Product  Inputs=*/  OutDataTypeStr=single
  Flux_d Lookup Table : Lookup_n-D  BreakpointsForDimension1=d_current_q_Flux  BreakpointsForDimension2=q_current_q_Flux  BreakpointsForDimension3=[5, 7]  Table=Flux_d  ExtrapMethod=Clip  UseLastTableValue=on  InternalRulePriority=Speed  OutDataTypeStr=Inherit: Inherit from 'Table data'  RndMeth=Simplest
      settings: InputPortMap=u0,u1
  Flux_q Lookup Table : Lookup_n-D  BreakpointsForDimension1=d_current_q_Flux  BreakpointsForDimension2=q_current_q_Flux  BreakpointsForDimension3=[5, 7]  Table=Flux_q  ExtrapMethod=Clip  UseLastTableValue=on  InternalRulePriority=Speed  OutDataTypeStr=Inherit: Inherit from 'Table data'  RndMeth=Simplest
      settings: InputPortMap=u0,u1
  Ldd Lookup Table : Lookup_n-D  BreakpointsForDimension1=d_current_q_Flux  BreakpointsForDimension2=q_current_q_Flux  BreakpointsForDimension3=[5, 7]  Table=Ldd  ExtrapMethod=Clip  UseLastTableValue=on  InternalRulePriority=Speed  OutDataTypeStr=Inherit: Inherit from 'Table data'  RndMeth=Simplest
      settings: InputPortMap=u0,u1
  Ldq Lookup Table2 : Lookup_n-D  BreakpointsForDimension1=d_current_q_Flux  BreakpointsForDimension2=q_current_q_Flux  BreakpointsForDimension3=[5, 7]  Table=Ldq  ExtrapMethod=Clip  UseLastTableValue=on  InternalRulePriority=Speed  OutDataTypeStr=Inherit: Inherit from 'Table data'  RndMeth=Simplest
      settings: InputPortMap=u0,u1
  Lqd Lookup Table1 : Lookup_n-D  BreakpointsForDimension1=d_current_q_Flux  BreakpointsForDimension2=q_current_q_Flux  BreakpointsForDimension3=[5, 7]  Table=Lqd  ExtrapMethod=Clip  UseLastTableValue=on  InternalRulePriority=Speed  OutDataTypeStr=Inherit: Inherit from 'Table data'  RndMeth=Simplest
      settings: InputPortMap=u0,u1
  Lqq Lookup Table : Lookup_n-D  BreakpointsForDimension1=d_current_q_Flux  BreakpointsForDimension2=q_current_q_Flux  BreakpointsForDimension3=[5, 7]  Table=Lqq  ExtrapMethod=Clip  UseLastTableValue=on  InternalRulePriority=Speed  OutDataTypeStr=Inherit: Inherit from 'Table data'  RndMeth=Simplest
      settings: InputPortMap=u0,u1
  Product{2..4,9,11..13} (7 alike) : Product  OutDataTypeStr=single
  Subsystem : Subsystem
  Subsystem1 : Subsystem
  Sum3 : Sum  Inputs=|+--+
  Sum4 : Sum  Inputs=|---+
  Unit Delay : UnitDelay  SampleTime=-1  HasFrameUpgradeWarning=on
  Unit Delay1 : UnitDelay  SampleTime=-1  HasFrameUpgradeWarning=on
  I_d1 : Outport
  psi_d1 : Outport  Port=2
  psi_q1 : Outport  Port=3
  I_q1 : Outport  Port=4
  wires:
  omega_mech1/1 -> Product13/1  "u_q"
  Flux_d Lookup Table/1 -> psi_d1/1, Product2/1  "psi_d"
  Lqq Lookup Table/1 -> Divide1/2  "Lqq"
  Ldd Lookup Table/1 -> Divide/1  "Ldd"
  Flux_q Lookup Table/1 -> Product3/2, psi_q1/1  "psi_q"
  Product11/1 -> Sum4/1
  Product12/1 -> Sum3/3
  Ldq Lookup Table2/1 -> Product12/1  "Ldq"
  Lqd Lookup Table1/1 -> Product11/2  "Lqd"
  Unit Delay1/1 -> Product12/2
  Unit Delay/1 -> Product11/1
  Product2/1 -> Sum4/2  "psi_d*omega_ell"
  Product4/1 -> Sum3/2
  Product3/1 -> Sum3/4  "psi_q*omega_ell"
  Subsystem1/1(outt) -> Product9/1, Lqd Lookup Table1/2, Ldq Lookup Table2/2, Flux_d Lookup Table/2, Flux_q Lookup Table/2, I_q1/1, Lqq Lookup Table/2, Ldd Lookup Table/2  "i_q"
  Subsystem/1(outt) -> I_d1/1, Flux_q Lookup Table/1, Flux_d Lookup Table/1, Product4/2, Ldd Lookup Table/1, Lqq Lookup Table/1, Ldq Lookup Table2/1, Lqd Lookup Table1/1  "id"
  R2/1 -> Product4/1, Product9/2
  u_d1/1 -> Sum3/1
  reset1/1 -> Subsystem1/2(reset), Subsystem/2(reset)
  Product9/1 -> Sum4/3
  Sum3/1 -> Divide/2
  Divide/1 -> Subsystem/1(in), Unit Delay/1  "did/dt"
  Product13/1 -> Product2/2, Product3/1
  polepairs1/1 -> Product13/2
  Divide1/1 -> Subsystem1/1(in), Unit Delay1/1  "diq/dt"
  u_q1/1 -> Sum4/4
  Sum4/1 -> Divide1/1

== system gm_uz_pmsm_model_6LUT_pd_vnl/uz_pmsm_model_6LUT_vnl/torque_calculation ==
  I_d : Inport
  psi_d : Inport  Port=2
  psi_q : Inport  Port=3
  polepairs : Inport  Port=4
  I_q : Inport  Port=5
  Factor : Gain  Gain=(3/2)
  Product2 : Product
  Product3 : Product
  Product9 : Product
  Sum3 : Sum  Inputs=-|+
  M_Mi : Outport
  wires:
  Factor/1 -> Product9/1  "M_Mi"
  polepairs/1 -> Product9/2
  Product9/1 -> M_Mi/1  "M_Mi"
  I_q/1 -> Product3/2
  I_d/1 -> Product2/1
  psi_d/1 -> Product3/1
  psi_q/1 -> Product2/2
  Product2/1 -> Sum3/1
  Product3/1 -> Sum3/2
  Sum3/1 -> Factor/1

== system gm_uz_pmsm_model_6LUT_pd_vnl/Compare/Assert_outputs/RelErrCheck ==
  In1 : Inport
  In2 : Inport  Port=2
  "RelativeErrorCheck " : MATLAB Function  TreatAsAtomicUnit=on
  Out1 : Outport  VectorParamsAs1DForOutWhenUnconnected=off
  wires:
  "RelativeErrorCheck "/1(y) -> Out1/1
  In1/1 -> "RelativeErrorCheck "/1(P)
  In2/1 -> "RelativeErrorCheck "/2(R)

== system gm_uz_pmsm_model_6LUT_pd_vnl/Current_Controller/Entkopplungen/Lineare_Entkopplung ==
  i_d : Inport
  i_q : Inport  Port=2
  omega_m : Inport  Port=3
  Constant1 : Constant  Value=psi_pm  SampleTime=-1
  Gain : Gain  Gain=L_q
  Gain1 : Gain  Gain=L_d
  Gain2 : Gain  Gain=polepair
  Product : Product
  Product1 : Product
  Sum6 : Sum  Inputs=|++
  u_d : Outport
  u_q : Outport  Port=2
  wires:
  omega_m/1 -> Gain2/1
  Sum6/1 -> Product1/1
  Product/1 -> u_d/1
  i_d/1 -> Gain1/1
  Constant1/1 -> Sum6/2
  i_q/1 -> Gain/1
  Product1/1 -> u_q/1
  Gain1/1 -> Sum6/1
  Gain2/1 -> Product1/2, Product/2
  Gain/1 -> Product/1

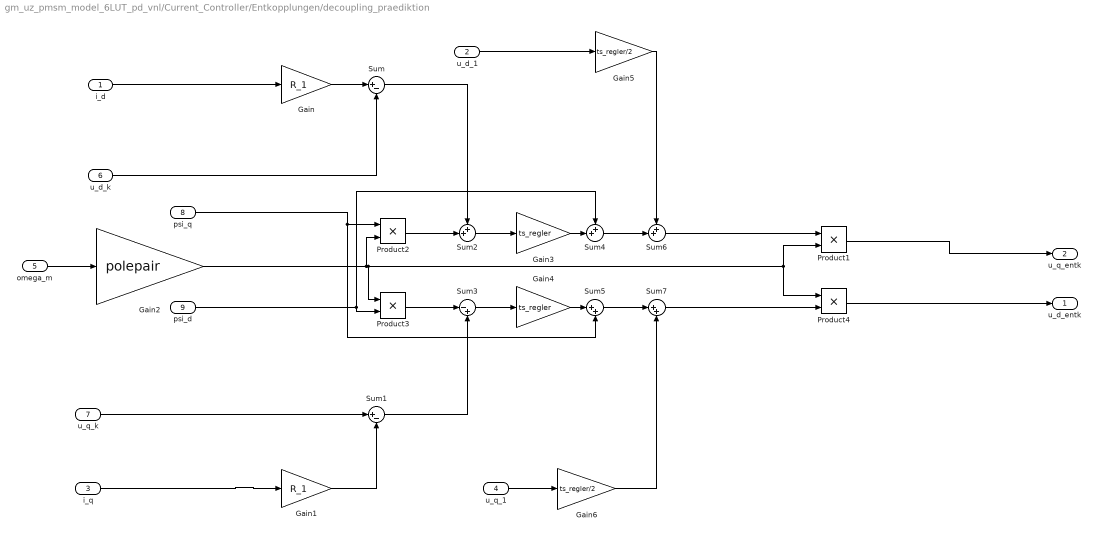
== system gm_uz_pmsm_model_6LUT_pd_vnl/Current_Controller/Entkopplungen/decoupling_praediktion ==
  i_d : Inport
  u_d_1 : Inport  Port=2
  i_q : Inport  Port=3
  u_q_1 : Inport  Port=4
  omega_m : Inport  Port=5
  u_d_k : Inport  Port=6
  u_q_k : Inport  Port=7
  psi_q : Inport  Port=8
  psi_d : Inport  Port=9
  Gain : Gain  Gain=R_1
  Gain1 : Gain  Gain=R_1
  Gain2 : Gain  Gain=polepair
  Gain3 : Gain  Gain=ts_regler
  Gain4 : Gain  Gain=ts_regler
  Gain5 : Gain  Gain=ts_regler/2
  Gain6 : Gain  Gain=ts_regler/2
  Product{1..4} (4 alike) : Product
  Sum : Sum  Inputs=|+-
  Sum1 : Sum  Inputs=|+-
  Sum2 : Sum  Inputs=++|
  Sum3 : Sum  Inputs=|-+
  Sum4 : Sum  Inputs=++|
  Sum5 : Sum  Inputs=|++
  Sum6 : Sum  Inputs=++|
  Sum7 : Sum  Inputs=|++
  u_d_entk : Outport
  u_q_entk : Outport  Port=2
  wires:
  psi_q/1 -> Sum5/2, Product2/1
  psi_d/1 -> Product3/2, Sum4/1
  Gain2/1 -> Product1/2, Product4/1, Product3/1, Product2/2
  u_d_k/1 -> Sum/2
  Gain/1 -> Sum/1
  u_q_k/1 -> Sum1/1
  Gain1/1 -> Sum1/2
  Product3/1 -> Sum3/1
  Product2/1 -> Sum2/2
  Sum/1 -> Sum2/1
  Sum1/1 -> Sum3/2
  Sum3/1 -> Gain4/1
  Sum2/1 -> Gain3/1
  Gain3/1 -> Sum4/2
  Gain4/1 -> Sum5/1
  u_d_1/1 -> Gain5/1
  Sum4/1 -> Sum6/2
  u_q_1/1 -> Gain6/1
  Gain5/1 -> Sum6/1
  Sum5/1 -> Sum7/1
  Gain6/1 -> Sum7/2
  Sum6/1 -> Product1/1
  Sum7/1 -> Product4/2
  omega_m/1 -> Gain2/1
  i_d/1 -> Gain/1
  i_q/1 -> Gain1/1
  Product1/1 -> u_q_entk/1
  Product4/1 -> u_d_entk/1

== system gm_uz_pmsm_model_6LUT_pd_vnl/Current_Controller/Entkopplungen/static_nonlinear_entkopplung ==
  psi_d : Inport
  psi_q : Inport  Port=2
  omega_m : Inport  Port=3
  Gain2 : Gain  Gain=polepair
  Product : Product
  Product1 : Product
  Scope : Scope  NumInputPorts=2
  u_d : Outport
  u_q : Outport  Port=2
  wires:
  psi_q/1 -> Product/1  "psi_q_LUT"
  Gain2/1 -> Product1/2, Product/2
  Product1/1 -> Scope/1, u_q/1
  Product/1 -> Scope/2, u_d/1
  psi_d/1 -> Product1/1  "psi_d_LUT"
  omega_m/1 -> Gain2/1

== system gm_uz_pmsm_model_6LUT_pd_vnl/Current_Controller/Entkopplungen/static_nonlinear_entkopplung1 ==
  psi_d : Inport
  psi_q : Inport  Port=2
  omega_m : Inport  Port=3
  Gain2 : Gain  Gain=polepair
  Product : Product
  Product1 : Product
  Scope : Scope  NumInputPorts=2
  u_d : Outport
  u_q : Outport  Port=2
  wires:
  psi_q/1 -> Product/1  "psi_q_LUT"
  Gain2/1 -> Product1/2, Product/2
  Product1/1 -> Scope/1, u_q/1
  Product/1 -> Scope/2, u_d/1
  psi_d/1 -> Product1/1  "psi_d_LUT"
  omega_m/1 -> Gain2/1

== system gm_uz_pmsm_model_6LUT_pd_vnl/uz_pmsm_model_6LUT_vnl/mechanical_system/integrator1 ==
  reset : Inport
  in : Inport  Port=2
  Delay1 : Delay  DelayLength=1  ExternalReset=Level
      settings: InputPortMap=u0,r5
  Gain : Gain  Gain=ts  OutDataTypeStr=single
  Sum3 : Sum  Inputs=|++  OutDataTypeStr=single
  outt : Outport
  wires:
  Delay1/1 -> outt/1, Sum3/2
  Sum3/1 -> Delay1/1
  reset/1 -> Delay1/2
  Gain/1 -> Sum3/1
  in/1 -> Gain/1

== system gm_uz_pmsm_model_6LUT_pd_vnl/uz_pmsm_model_6LUT_vnl/pmsm/Subsystem ==
  in : Inport
  reset : Inport  Port=2
  Delay1 : Delay  DelayLength=1  ExternalReset=Level
      settings: InputPortMap=u0,r5
  Gain7 : Gain  Gain=ts  OutDataTypeStr=single
  Sum5 : Sum  Inputs=|++  OutDataTypeStr=single
  outt : Outport
  wires:
  Gain7/1 -> Sum5/1  "u_d"
  Sum5/1 -> Delay1/1
  Delay1/1 -> Sum5/2, outt/1
  reset/1 -> Delay1/2
  in/1 -> Gain7/1

== system gm_uz_pmsm_model_6LUT_pd_vnl/uz_pmsm_model_6LUT_vnl/pmsm/Subsystem1 ==
  in : Inport
  reset : Inport  Port=2
  Delay1 : Delay  DelayLength=1  ExternalReset=Level
      settings: InputPortMap=u0,r5
  Gain7 : Gain  Gain=ts  OutDataTypeStr=single
  Sum5 : Sum  Inputs=|++  OutDataTypeStr=single
  outt : Outport
  wires:
  Gain7/1 -> Sum5/1  "u_d"
  Sum5/1 -> Delay1/1
  Delay1/1 -> Sum5/2, outt/1
  reset/1 -> Delay1/2
  in/1 -> Gain7/1

== matlab function gm_uz_pmsm_model_6LUT_pd_vnl/Compare/Assert_outputs/RelErrCheck/RelativeErrorCheck  ==
  data: P input; y output; R input; ToleranceValue parameter double
% Check if the relative error of R with respect to P is below
% ToleranceValue
% P, R are floating-point
function y = relErrCheck(P,R, ToleranceValue)
    tol = ToleranceValue;
    sz = numel(P);
    assert(sz == numel(R), 'Inputs P and R have different sizes.');
    y = false(1, sz);

    for ii=1:sz
        if (isnan(P(ii)) || isnan(R(ii)))
            if (isnan(P(ii)) && isnan(R(ii)))
                y(ii) = true;
            end
        elseif (isinf(P(ii)) || isinf(R(ii)))
            y(ii) = (P(ii) == R(ii));
        elseif (P(ii) == 0)
            y(ii) = (R(ii) == 0);
        else
            absdiff = abs(P(ii) - R(ii));
            relerr = absdiff/abs(P(ii));
            y(ii) = (relerr <= tol);
        end
    end
end
